simulink model "LaneDepartureDetection"  (R2024b)
settings: Solver=FixedStepAuto  StartTime=0.0  StopTime=25  FixedStep=0.001  RelTol=1e-3
values from neighbouring files (symbols this model uses):
  AmplitudeOfSineWaveThatMatchesMaxCurvatureOfInterstate = ((wavelengthOfSineWaveInMeters^2 * curvatureOfInterstate) / (4 * pi^2))    (= 2.71264458036)    [LaneDepartureDetectionWorkspace.m]
  distanceFromCenterlineToEdgeOfLaneInMeters = widthOfLaneInMeters / 2    (= 1.8288)    [LaneDepartureDetectionWorkspace.m]
  heightOfCenterOfGravityInMeters = 0.1    [LaneDepartureDetectionWorkspace.m]
  massOfVehicleInKilograms = 1500    [LaneDepartureDetectionWorkspace.m]
  meterToMillimeterConversionFactor = 1000    [LaneDepartureDetectionWorkspace.m]
  seventyMilesPerHourInMetersPerSecond = seventyMilesPerHour * milesPerHourToMetersPerSecondConversionFactor    (= 31.2928)    [LaneDepartureDetectionWorkspace.m]
  springDampingInNewtonMeterSecondsPerMeter = 2000    [LaneDepartureDetectionWorkspace.m]
  steeringFrequencySmoothingCutoffInRadiansPerSecond = 0.5    [LaneDepartureDetectionWorkspace.m]
  tenDegreesInRadians = tenDegrees * degreesToRadiansConversionFactor    (= 0.349066)    [LaneDepartureDetectionWorkspace.m]
  thirtyDegreesInRadians = thirtyDegrees * degreesToRadiansConversionFactor    (= 0.523599)    [LaneDepartureDetectionWorkspace.m]
  typicalCarTrackWidthInMeters = typicalCarTrackWidthInFeet * footToMeterConversionFactor    (= 1.524)    [LaneDepartureDetectionWorkspace.m]
  typicalCarWheelbaseInMeters = typicalCarWheelbaseInFeet * footToMeterConversionFactor    (= 2.8956)    [LaneDepartureDetectionWorkspace.m]
  widthOfLaneInMeters = widthOfLaneInFeet * footToMeterConversionFactor    (= 3.6576)    [LaneDepartureDetectionWorkspace.m]
libraries: fl_lib x5, nesl_utility x3, cstblocks x1
settings Model: Creator=jpeters  LastModifiedBy=jpeters

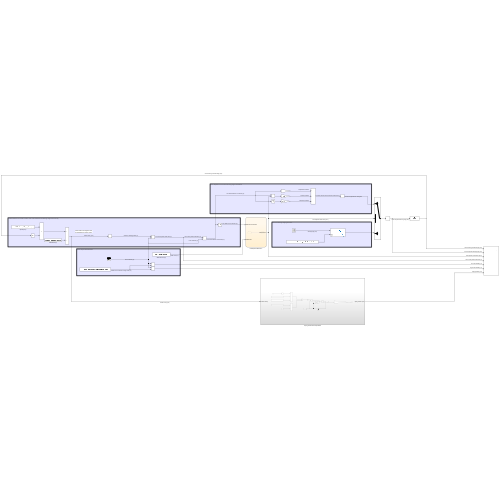
[thumbnail: Simulink's stored preview of the top-level diagram]
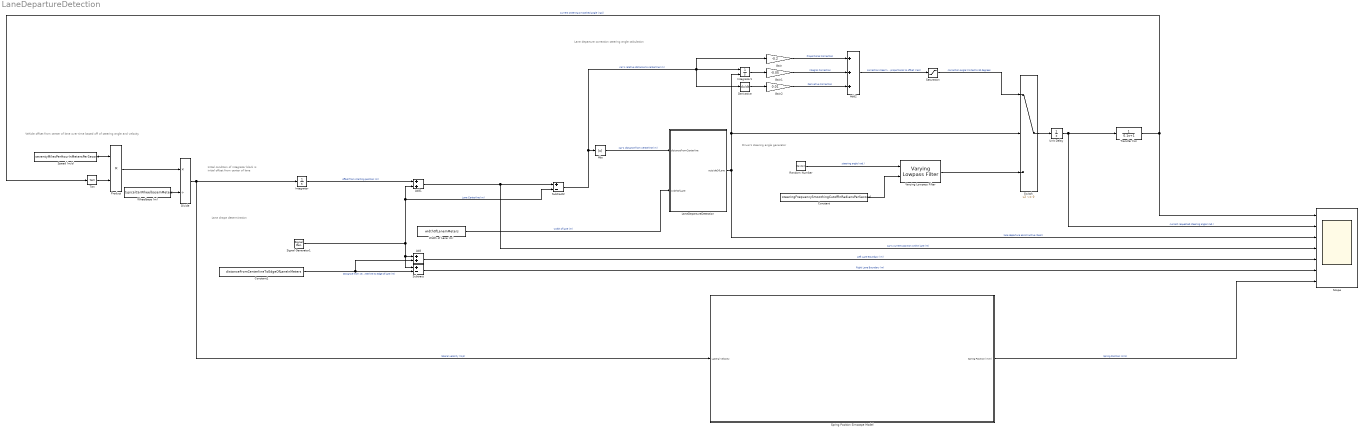
== system LaneDepartureDetection ==
  note: Driver's steering angle generator
  note: Lane departure correction steering angle calculation
  note: Lane shape determination
  note: Vehicle offset from center of lane over time based off of steering angle and velocity
  note: Initial condition of integrator block is initial offset from center of lane
  Abs : Abs  SaturateOnIntegerOverflow=off
  Add : Sum
  Add1 : Sum
  Add2 : Sum  Inputs=+++
  Constant : Constant  Value=steeringFrequencySmoothingCutoffInRadiansPerSecond
  Constant1 : Constant  Value=distanceFromCenterlineToEdgeOfLaneInMeters
  Derivative : Derivative
  Divide : Product  Inputs=*/
  Gain : Gain  Gain=-0.2
  Gain1 : Gain  Gain=-0.05
  Gain2 : Gain  Gain=0.01
  Integrator : Integrator
  Integrator1 : Integrator  ExternalReset=rising
  LaneDepartureDetection : Stateflow chart  TreatAsAtomicUnit=on
  Product : Product
  Random Number : RandomNumber  Variance=tenDegreesInRadians  Seed=10  SampleTime=0.1
  Saturation : Saturate  UpperLimit=thirtyDegreesInRadians  LowerLimit=-thirtyDegreesInRadians
  Scope : Scope  NumInputPorts=7
  Signal Generator1 : SignalGenerator  Amplitude=AmplitudeOfSineWaveThatMatchesMaxCurvatureOfInterstate  Frequency=0.1
  Speed (m/s) : Constant  Value=seventyMilesPerHourInMetersPerSecond
  Spring Position Simscape Model : Subsystem
  Subtract : Sum  Inputs=+-
  Subtract2 : Sum  Inputs=+-
  Switch : Switch  Criteria=u2 ~= 0  Threshold=1  SaturateOnIntegerOverflow=off  InputSameDT=off
  Tan : Trigonometry  Operator=tan
  Transfer Fcn : TransferFcn  Denominator=[0.1 1]
  Unit Delay : UnitDelay  SampleTime=-1  HasFrameUpgradeWarning=on
  Varying Lowpass Filter : cstblocks/Linear Parameter Varying/Varying Lowpass Filter  N=1
  Wheelbase (m) : Constant  Value=typicalCarWheelbaseInMeters
  Width of Lane (m) : Constant  Value=widthOfLaneInMeters
  wires:
  Speed (m/s)/1 -> Product/1
  Random Number/1 -> Varying Lowpass Filter/1  "steering angle (rad.)"
  Wheelbase (m)/1 -> Divide/2
  Tan/1 -> Product/2
  Product/1 -> Divide/1
  Divide/1 -> Spring Position Simscape Model/1(Lateral Velocity), Integrator/1  "lateral velocity (m/s)"
  Signal Generator1/1 -> Subtract/1, Add/1, Subtract2/2, Add1/2  "Lane Centerline (m)"
  Add/1 -> Scope/5  "Left Lane Boundary (m)"
  Width of Lane (m)/1 -> LaneDepartureDetection/2(widthOfLane)  "width of lane (m)"
  Constant1/1 -> Add/2, Subtract/2  "Distance from centerline to edge of lane (m)"
  Subtract/1 -> Scope/6  "Right Lane Boundary (m)"
  LaneDepartureDetection/1(outsideOfLane) -> Switch/2, Integrator1/2, Scope/3  "lane departure assist active (bool.)"
  Switch/1 -> Unit Delay/1
  Add2/1 -> Saturation/1  "correction steering angle proportional to offset (rad.)"
  Saturation/1 -> Switch/1  "correction angle limited to 30 degrees"
  Integrator/1 -> Add1/1  "offset from starting position (m)"
  Gain/1 -> Add2/1  "Proportional Correction"
  Integrator1/1 -> Gain1/1
  Derivative/1 -> Gain2/1
  Gain1/1 -> Add2/2  "Integral Correction"
  Gain2/1 -> Add2/3  "Derivative Correction"
  Add1/1 -> Scope/4, Subtract2/1  "car's current position within lane (m)"
  Subtract2/1 -> Gain/1, Derivative/1, Integrator1/1, Abs/1  "car's relative distance to centerline (m)"
  Abs/1 -> LaneDepartureDetection/1(distanceFromCenterline)  "car's distance from centerline (m)"
  Transfer Fcn/1 -> Scope/1, Tan/1  "current steering smoothed angle (rad.)"
  Unit Delay/1 -> Scope/2, Transfer Fcn/1  "current requested steering angle (rad.)"
  Varying Lowpass Filter/1 -> Switch/3
  Spring Position Simscape Model/1(Spring Position (mm)) -> Scope/7  "Spring Position (mm)"
  Constant/1 -> Varying Lowpass Filter/2

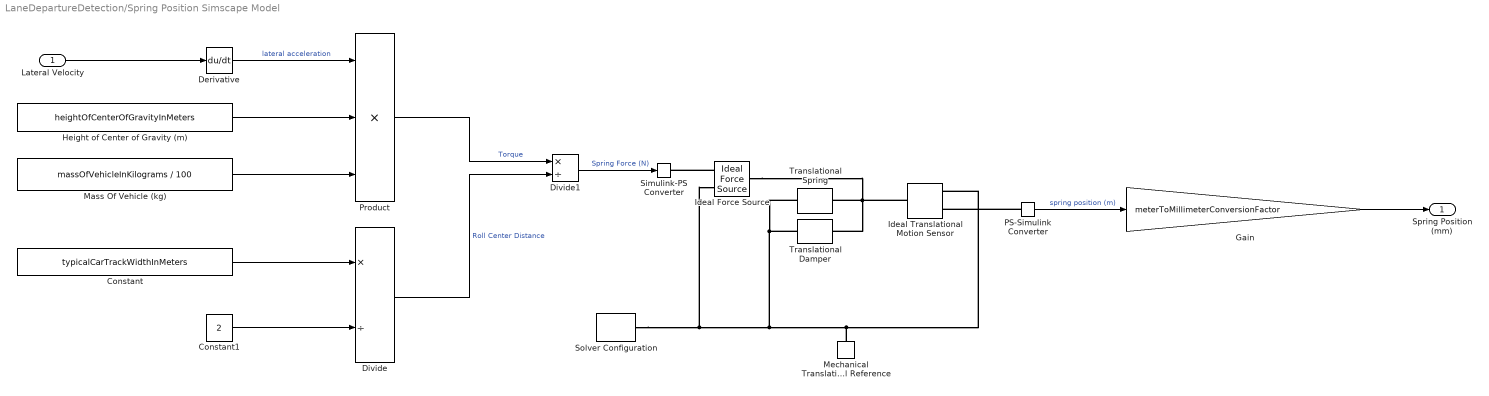
== system LaneDepartureDetection/Spring Position Simscape Model ==
  Lateral Velocity : Inport
  Constant : Constant  Value=typicalCarTrackWidthInMeters
  Constant1 : Constant  Value=2
  Derivative : Derivative
  Divide : Product  Inputs=*/
  Divide1 : Product  Inputs=*/
  Gain : Gain  Gain=meterToMillimeterConversionFactor
  Height of Center of Gravity (m) : Constant  Value=heightOfCenterOfGravityInMeters
  Ideal Force Source : fl_lib/Mechanical/Mechanical Sources/Ideal Force Source
  Ideal Translational Motion Sensor : fl_lib/Mechanical/Mechanical Sensors/Ideal Translational Motion Sensor  reference=foundation.enum.MeasurementReference.difference  acceleration_port=false  velocity_port=false  position_port=true  offset=0 m
      settings: InternalSimscapePortConfiguration="{\"Bottom\":[],\"Left\":[{\"id\":\"R\",\"label\":\"R\",\"type\":\"foundation.mechanical.translational.translational\"}],\"Right\":[{\"id\":\"C\",\"label\":\"C\",\"type\":\"foundation.mechanical.translational.translational\"},{\"id\":\"P\",\"label\":\"P\",\"type\":\"output\"}],\"Top\":[]}"
  Mass Of Vehicle (kg) : Constant  Value=massOfVehicleInKilograms / 100
  Mechanical Translational Reference : fl_lib/Mechanical/Translational Elements/Mechanical Translational Reference
  PS-Simulink Converter : nesl_utility/PS-Simulink Converter  PhysicalDomain=network_engine_domain  SubClassName=ps_output  LeftPortType=input  RightPortType=output  PseudoPeriodic=off  Frequencies=[]  VectorFormat=inherit  Unit=inherit  AffineConversion=off
  Product : Product  Inputs=3
  Simulink-PS Converter : nesl_utility/Simulink-PS Converter  PhysicalDomain=network_engine_domain  SubClassName=ps_input  LeftPortType=input  RightPortType=output  PseudoPeriodic=off  Frequencies=[]  NoiseDistribution=none  NoiseParameters=[]  Unit=1  AffineConversion=off  FilteringAndDerivatives=provide  SimscapeFilterOrder=1  InputFilterTimeConstant=0.001  UdotUserProvided=0
  Solver Configuration : nesl_utility/Solver Configuration  PhysicalDomain=network_engine_domain  SubClassName=solver  LeftPortType=input  RightPortType=generic  Tones=[]  Harmonics=[]  SimulateNoise=off  Profile=off  UseLocalSampling=off  EnableSwitchedLinearOptims=on  FrequencyDomain=off  UseCCode=off  RelTol=0.001  AbsTol=0.001  MinStep=1e-09  ToWorkspace=off  RevertToSquareIcSolve=off  NumHomotopyIterations=100  PhasorMode=off  PhasorModeNumHarmonics=1  ConsistencySolver=NEWTON_XTOL_AFTER_FTOL  IndexReductionMethod=DerivativeReplacement  DoDC=off  ResidualTolerance=1e-09  ConsistencyTolSource=GLOBAL  ConsistencyAbsTol=0.001  ConsistencyRelTol=0.001  ConsistencyTolFactor=0.001  UseLocalSolver=off  LocalSolverChoice=NE_BACKWARD_EULER_ADVANCER  ResolveIndetEquations=on  FunctionEvalNumThread=1  LocalSolverSampleTime=0.001  DoFixedCost=off  MaxNonlinIter=3  MaxModeIter=2  ComputeImpulses=off  ImpulseIterations=2  LinearAlgebra=auto  LinearAlgebraNumThread=0  EquationFormulation=NE_TIME_EF  DelaysMemoryBudget=1024  AutomaticFiltering=on  FilteringTimeConstant=0.001  PartitionStorageMethod=AS_NEEDED  PartitionMemoryBudget=1024  PartitionMethod=ROBUST  MultibodyUseLocalSolver=off  MultibodyLocalSolverChoice=ODE1  MultibodyLocalSolverSampleTime=0.001
  Translational Damper : fl_lib/Mechanical/Translational Elements/Translational Damper  D=springDampingInNewtonMeterSecondsPerMeter N*s/m  v_specify=off  v_priority=None  v=0 m/s  v_nominal_specify=off  v_nominal_value=1  v_nominal_unit=m/s  f_specify=off  f_priority=None  f=0 N  f_nominal_specify=off  f_nominal_value=1  f_nominal_unit=N
  Translational Spring : fl_lib/Mechanical/Translational Elements/Translational Spring  spr_rate=springStiffnessInNewtonMetersPerMeter N/m  v_specify=off  v_priority=None  v=0 m/s  v_nominal_specify=off  v_nominal_value=1  v_nominal_unit=m/s  f_specify=off  f_priority=None  f=0 N  f_nominal_specify=off  f_nominal_value=1  f_nominal_unit=N  x_specify=off  x_priority=High  x=0 m  x_nominal_specify=off  x_nominal_value=1  x_nominal_unit=m
  Spring Position (mm) : Outport
  wires:
  Lateral Velocity/1 -> Derivative/1
  Height of Center of Gravity (m)/1 -> Product/2
  Product/1 -> Divide1/1  "Torque"
  Constant/1 -> Divide/1
  Constant1/1 -> Divide/2
  Divide/1 -> Divide1/2  "Roll Center Distance"
  Divide1/1 -> Simulink-PS Converter/1  "Spring Force (N)"
  Derivative/1 -> Product/1  "lateral acceleration"
  Mass Of Vehicle (kg)/1 -> Product/3
  PS-Simulink Converter/1 -> Gain/1  "spring position (m)"
  Gain/1 -> Spring Position (mm)/1
  connections:
  Ideal Translational Motion Sensor/LConn1 -- Ideal Force Source/LConn1 -- Translational Damper/LConn1 -- Translational Spring/LConn1
  Ideal Force Source/RConn1 -- Simulink-PS Converter/RConn1
  PS-Simulink Converter/LConn1 -- Ideal Translational Motion Sensor/RConn2
  Solver Configuration/RConn1 -- Ideal Translational Motion Sensor/RConn1 -- Mechanical Translational Reference/LConn1 -- Translational Spring/RConn1 -- Translational Damper/RConn1 -- Ideal Force Source/RConn2

== stateflow chart LaneDepartureDetection/LaneDepartureDetection ==
  state WithinLane
    entry:
    outsideOfLane = false;
  state OutsideOfLane
    entry:
    outsideOfLane = true;
  (default) -> WithinLane
  WithinLane -> OutsideOfLane : [distanceFromCenterline >= (widthOfLane / 2)]
  OutsideOfLane -> WithinLane : [distanceFromCenterline <= (widthOfLane / 10)]
  data: outsideOfLane output; distanceFromCenterline input; widthOfLane input
